simulink model "si2_Fourierseries"  (R2021b)
settings: Solver=ode45  StartTime=-8  StopTime=8  MaxStep=0.01  RelTol=1e-3  EnableMultiTasking=on
settings Model: Creator=peter  LastModifiedBy=sar
settings SolverCC: AlgebraicLoopSolver=TrustRegion
settings DataIOCC: LimitDataPoints=on  SaveFormat=Array  SignalLoggingSaveFormat=ModelDataLogs  ReturnWorkspaceOutputs=off  SignalLoggingName=sigsOut
settings OptimizationCC: BooleanDataType=off  ExpressionDepthLimit=2147483647  LifeSpan=inf
settings DebuggingCC: SaveWithParameterizedLinksMsg=none  UnderspecifiedInitializationDetection=Classic  MergeDetectMultiDrivingBlocksExec=none  SignalResolutionControl=TryResolveAllWithWarning  MultiTaskDSMMsg=warning  MultiTaskCondExecSysMsg=none  FcnCallInpInsideContextMsg=warning  StateNameClashWarn=warning  SFUnexpectedBacktrackingDiag=warning  SFNoUnconditionalDefaultTransitionDiag=warning  SFMachineParentedDataDiag=warning  ArithmeticOperatorsInVariantConditions=warning
settings HardwareCC: ProdBitPerPointer=32  ProdBitPerSizeT=32  ProdBitPerPtrDiffT=32  ProdLargestAtomicFloat=None  ProdIntDivRoundTo=Undefined  ProdEndianess=Unspecified  ProdWordSize=32  ProdHWDeviceType=32-bit Generic  TargetUnknown=on
settings ModelReferenceCC: PropagateSignalLabelsOutOfModel=off
settings SFSimCC: SimUseLocalCustomCode=off  CustomCodeUndefinedFunction=UseInterfaceOnly
settings RTWCC: RTWUseLocalCustomCode=off
settings CodeAppCC: StateflowObjectComments=on
settings GRTTargetCC: TargetLangStandard=C89/C90 (ANSI)  CombineOutputUpdateFcns=off  GRTInterface=on
settings ConfigComp: CovMetricSettings=dw  CovSaveCumulativeToWorkspaceVar=on  CovSaveSingleToWorkspaceVar=on  CovExternalEMLEnable=off

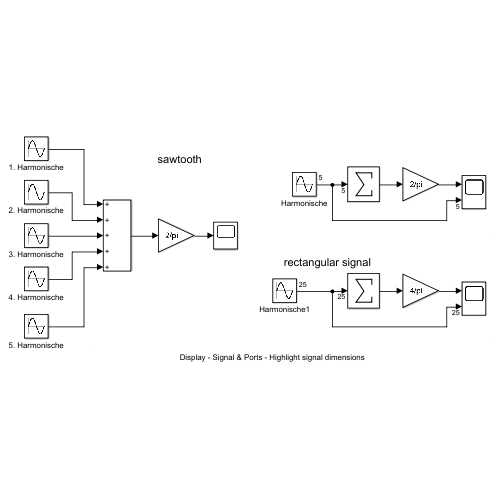
[thumbnail: Simulink's stored preview of the top-level diagram]
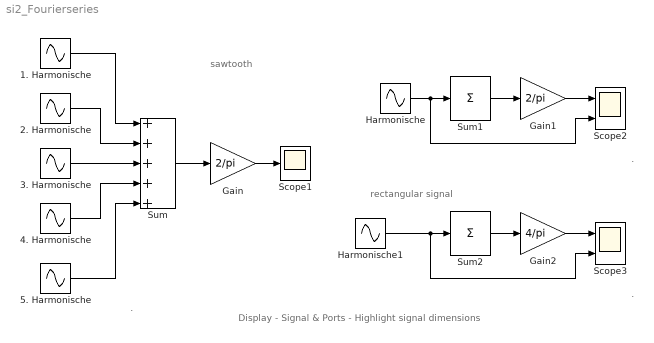
== system si2_Fourierseries ==
  note: Display - Signal & Ports - Highlight signal dimensions
  note: sawtooth
  note: .
  note: .
  note: .
  note: rectangular signal
  1. Harmonische : Sin  SampleTime=0
  2. Harmonische : Sin  Amplitude=1/2  Frequency=2  SampleTime=0
  3. Harmonische : Sin  Amplitude=1/3  Frequency=3  SampleTime=0
  4. Harmonische : Sin  Amplitude=1/4  Frequency=4  SampleTime=0
  5. Harmonische : Sin  Amplitude=1/5  Frequency=5  SampleTime=0
  Gain : Gain  Gain=2/pi  SaturateOnIntegerOverflow=on  OutDataTypeStr=Inherit: Same as input  ParamDataTypeStr=Inherit: Same as input
  Gain1 : Gain  Gain=2/pi  SaturateOnIntegerOverflow=on  OutDataTypeStr=Inherit: Same as input  ParamDataTypeStr=Inherit: Same as input
  Gain2 : Gain  Gain=4/pi  SaturateOnIntegerOverflow=on  OutDataTypeStr=Inherit: Same as input  ParamDataTypeStr=Inherit: Same as input
  Harmonische : Sin  Amplitude=1./(1:5)  Frequency=1:5  SampleTime=0
  Harmonische1 : Sin  Amplitude=1./(1:2:50)  Frequency=1:2:50  SampleTime=0
  Scope1 : Scope
  Scope2 : Scope  NumInputPorts=2
  Scope3 : Scope  NumInputPorts=2
  Sum : Sum  Inputs=5  SaturateOnIntegerOverflow=on
  Sum1 : Sum  Inputs=+  SaturateOnIntegerOverflow=on
  Sum2 : Sum  Inputs=+  SaturateOnIntegerOverflow=on
  wires:
  Gain/1 -> Scope1/1
  Sum/1 -> Gain/1
  3. Harmonische/1 -> Sum/3
  2. Harmonische/1 -> Sum/2
  1. Harmonische/1 -> Sum/1
  4. Harmonische/1 -> Sum/4
  5. Harmonische/1 -> Sum/5
  Sum1/1 -> Gain1/1
  Harmonische/1 -> Sum1/1, Scope2/2
  Gain1/1 -> Scope2/1
  Sum2/1 -> Gain2/1
  Harmonische1/1 -> Sum2/1, Scope3/2
  Gain2/1 -> Scope3/1
